simulink model "dc_motor_from_idtf"  (R2021a)
settings: Solver=VariableStepAuto  StartTime=0.0  StopTime=0.005  RelTol=1e-3
values from neighbouring files (symbols this model uses):
  Hs = struct([])    [test.m]
  T_l = T_l_range(1,i)    [Task1.m]    (also in Task2.m = 2.58; Task2b.m; Task3.m; Task4.m = T_l_range(1,k))
  V = 12    [Task1.m]    (also in Task2.m; Task2b.m; Task3.m; Task4.m = y(j,5))
settings Model: Creator=Usamat980  LastModifiedBy=Usamat980

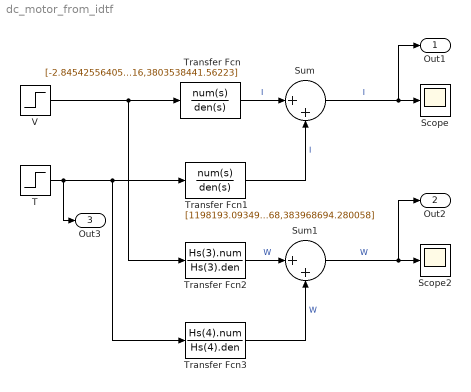
== system dc_motor_from_idtf ==
  Scope : Scope
  Scope2 : Scope
  Sum : Sum  Inputs=|++
  Sum1 : Sum  Inputs=|++
  T : Step  Time=0  After=T_l  SampleTime=0
  Transfer Fcn : TransferFcn  Numerator=[-2.84542556405772,951074.987439422]  Denominator=[1,103156.528746716,3803538441.56223]
  Transfer Fcn1 : TransferFcn  Numerator=[1198193.09349200,1397729262.00037]  Denominator=[1,88571.9182858268,383968694.280058]
  Transfer Fcn2 : TransferFcn  Numerator=Hs(3).num  Denominator=Hs(3).den
  Transfer Fcn3 : TransferFcn  Numerator=Hs(4).num  Denominator=Hs(4).den
  V : Step  Time=0  After=V  SampleTime=0
  Out1 : Outport
  Out2 : Outport  Port=2
  Out3 : Outport  Port=3
  wires:
  V/1 -> Transfer Fcn2/1, Transfer Fcn/1
  T/1 -> Out3/1, Transfer Fcn1/1, Transfer Fcn3/1
  Sum/1 -> Out1/1, Scope/1  "I"
  Transfer Fcn/1 -> Sum/1  "I"
  Transfer Fcn1/1 -> Sum/2  "I"
  Transfer Fcn2/1 -> Sum1/1  "W"
  Sum1/1 -> Out2/1, Scope2/1  "W"
  Transfer Fcn3/1 -> Sum1/2  "W"
